simulink model "ADCtoDACloopback"  (R2015b)
settings: Solver=VariableStepAuto  StartTime=0.0  StopTime=10.0  RelTol=1e-3
undefined symbols (not defined in the file): AXI4, fClk, Lite
libraries: xbsIndex_r4 x115
settings Model: Creator=sebek  LastModifiedBy=sebek

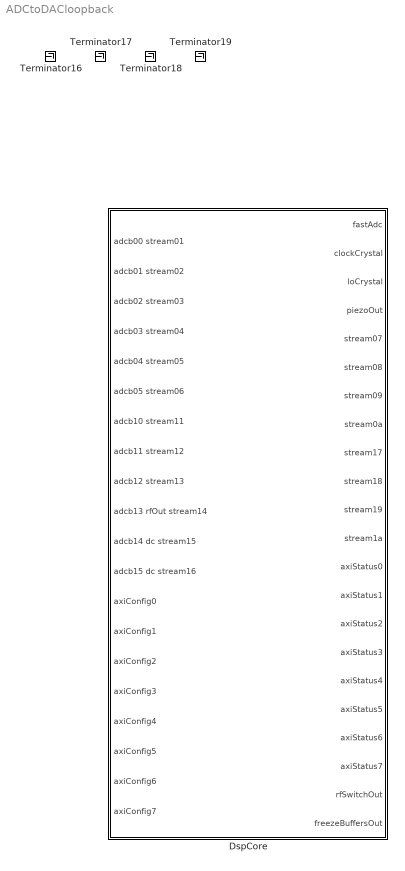
== system ADCtoDACloopback ==
  DspCore : Subsystem
  Terminator{16..19} (4 alike) : Terminator

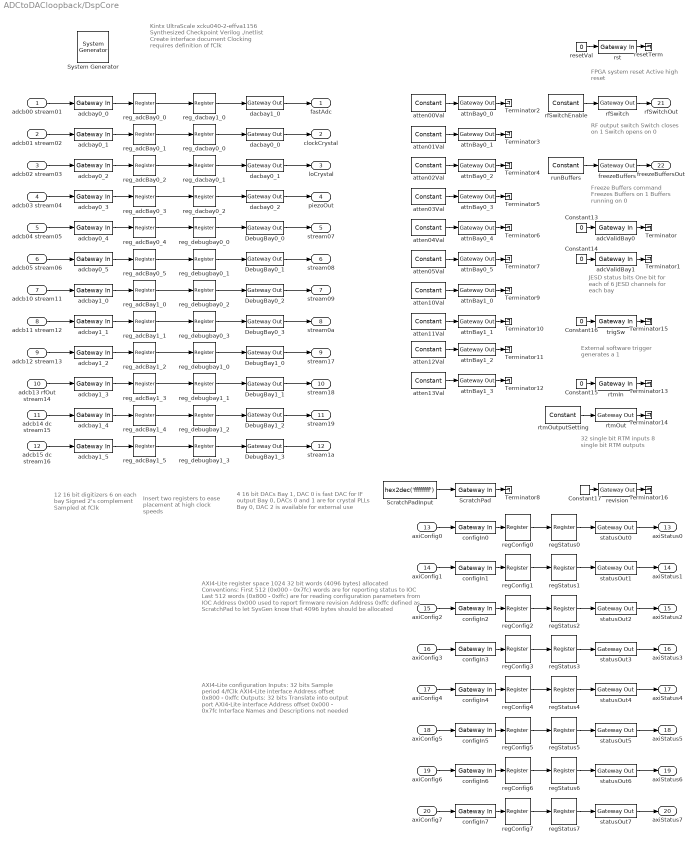
== system ADCtoDACloopback/DspCore ==
  note: AXI4-Lite configuration
      | Inputs:
      | 32 bits
      | Sample period 4/fClk
      | AXI4-Lite interface
      | Address offset 0x800 - 0xffc
      | Outputs:
      | 32 bits
      | Translate into output port
      | AXI4-Lite interface
      | Address offset 0x000 - 0x7fc
      | Interface Names and Descriptions not needed
  note: AXI4-Lite register space
      | 1024 32 bit words (4096 bytes) allocated
      | Conventions:
      | First 512 (0x000 - 0x7fc) words are for reporting status to IOC
      | Last 512 words (0x800 - 0xffc) are for reading configuration
      | parameters from IOC
      | Address 0x000 used to report firmware revision
      | Address 0xffc defined as ScratchPad to let SysGen know that
      | 4096 bytes should be allocated
  note: 32 single bit RTM inputs
      | 8 single bit RTM outputs
  note: External software trigger
      | generates a 1
  note: JESD status bits
      | One bit for each of
      | 6 JESD channels
      | for each bay
  note: RF output switch
      | Switch closes on 1
      | Switch opens on 0
  note: 4 16 bit DACs
      | Bay 1, DAC 0 is fast DAC for IF output
      | Bay 0, DACs 0 and 1 are for crystal PLLs
      | Bay 0, DAC 2 is available for external use
  note: Insert two registers
      | to ease placement
      | at high clock speeds
  note: 12 16 bit digitizers
      | 6 on each bay
      | Signed 2's complement
      | Sampled at fClk
  note: Kintx UltraScale xcku040-2-effva1156
      | Synthesized Checkpoint
      | Verilog
      | ./netlist
      | Create interface document
      | Clocking requires definition of fClk
  note: FPGA system reset
      | Active high reset
  note: Freeze Buffers command
      | Freezes Buffers on 1
      | Buffers running on 0
  adcb00 stream01 : Inport
  adcb01 stream02 : Inport  Port=2
  adcb02 stream03 : Inport  Port=3
  adcb03 stream04 : Inport  Port=4
  adcb04 stream05 : Inport  Port=5
  adcb05 stream06 : Inport  Port=6
  adcb10 stream11 : Inport  Port=7
  adcb11 stream12 : Inport  Port=8
  adcb12 stream13 : Inport  Port=9
  adcb13 rfOut stream14 : Inport  Port=10
  adcb14 dc stream15 : Inport  Port=11
  adcb15 dc stream16 : Inport  Port=12
  axiConfig0 : Inport  Port=13
  axiConfig1 : Inport  Port=14
  axiConfig2 : Inport  Port=15
  axiConfig3 : Inport  Port=16
  axiConfig4 : Inport  Port=17
  axiConfig5 : Inport  Port=18
  axiConfig6 : Inport  Port=19
  axiConfig7 : Inport  Port=20
  " System Generator" : xbsIndex_r4/ System Generator  Tag=genX  xilinxfamily=kintexu  part=xcku040  speed=-2-e  package=ffva1156  synthesis_tool=Vivado  clock_wrapper=Clock Enables  directory=./netlist  proj_type=Vivado  Synth_file=Vivado Synthesis Defaults  Impl_file=Vivado Implementation Defaults  testbench=off  simulink_period=1/fClk  sysclk_period=1/fClk*1e9  dcm_input_clock_period=10  incr_netlist=off  trim_vbits=Everywhere in SubSystem  dbl_ovrd=According to Block Masks  core_generation=According to Block Masks  run_coregen=off  deprecated_control=off  eval_field=0  block_type=sysgen
  Constant{13..16} (4 alike) : Constant  Value=0
  Constant17 : xbsIndex_r4/Constant  const=1  gui_display_data_type=Fixed-point  arith_type=Unsigned  n_bits=32  bin_pt=0  preci_type=Single  exp_width=8  frac_width=24  explicit_period=off  period=1  equ=P=C  opselect=C  inp2=PCIN>>17  opr=+  inp1=P  carry=CIN  dbl_ovrd=off  block_type=constant
  DebugBay0_{0..3} (4 alike) : xbsIndex_r4/Gateway Out  inherit_from_input=on  hdl_port=on  rows=1  columns=1  UseAsDAC=off  DACChannel='1'  interface=None  automatic_assignment=on  address_offset=hex2dec('00')  intf_name=''  intf_description=''  timing_constraint=None  locs_specified=off  LOCs={}  io_standard={}  block_type=gatewayout
  DebugBay1_{0..3} (4 alike) : xbsIndex_r4/Gateway Out  inherit_from_input=on  hdl_port=on  rows=1  columns=1  UseAsDAC=off  DACChannel='1'  interface=None  automatic_assignment=on  address_offset=hex2dec('00')  intf_name=''  intf_description=''  timing_constraint=None  locs_specified=off  LOCs={}  io_standard={}  block_type=gatewayout
  ScratchPad : xbsIndex_r4/Gateway In  gui_display_data_type=Fixed-point  arith_type=Unsigned  n_bits=32  bin_pt=0  preci_type=Single  exp_width=8  frac_width=24  rows=1  columns=1  quantization="Round  (unbiased: +/- Inf)"  overflow=Saturate  period=1  UseAsADC=off  ADCChannel='1'  interface=AXI4-Lite  automatic_assignment=off  address_offset=hex2dec('0ffc')  intf_name=''  intf_description=''  default_value=0  timing_constraint=None  locs_specified=off  LOCs={}  io_standard={}  inherit_from_input=off  hdl_port=on  dbl_ovrd=off  block_type=gatewayin
  ScratchPadInput : Constant  Value=hex2dec('ffffffff')  OutDataTypeStr=uint32
  Terminator{,1..16} (17 alike) : Terminator
  adcValidBay0 : xbsIndex_r4/Gateway In  gui_display_data_type=Fixed-point  arith_type=Unsigned  n_bits=6  bin_pt=0  preci_type=Single  exp_width=8  frac_width=24  rows=1  columns=1  quantization="Round  (unbiased: +/- Inf)"  overflow=Saturate  period=1/fClk  UseAsADC=off  ADCChannel='1'  interface=None  automatic_assignment=on  address_offset=hex2dec('00')  intf_name=''  intf_description=''  default_value=0  timing_constraint=None  locs_specified=off  LOCs={}  io_standard={}  inherit_from_input=off  hdl_port=on  dbl_ovrd=off  block_type=gatewayin
  adcValidBay1 : xbsIndex_r4/Gateway In  gui_display_data_type=Fixed-point  arith_type=Unsigned  n_bits=6  bin_pt=0  preci_type=Single  exp_width=8  frac_width=24  rows=1  columns=1  quantization="Round  (unbiased: +/- Inf)"  overflow=Saturate  period=1/fClk  UseAsADC=off  ADCChannel='1'  interface=None  automatic_assignment=on  address_offset=hex2dec('00')  intf_name=''  intf_description=''  default_value=0  timing_constraint=None  locs_specified=off  LOCs={}  io_standard={}  inherit_from_input=off  hdl_port=on  dbl_ovrd=off  block_type=gatewayin
  adcbay0_{0..5} (6 alike) : xbsIndex_r4/Gateway In  gui_display_data_type=Fixed-point  arith_type="Signed  (2's comp)"  n_bits=16  bin_pt=0  preci_type=Single  exp_width=8  frac_width=24  rows=1  columns=1  quantization="Round  (unbiased: +/- Inf)"  overflow=Saturate  period=1/fClk  UseAsADC=off  ADCChannel='1'  interface=None  automatic_assignment=on  address_offset=hex2dec('00')  intf_name=''  intf_description=''  default_value=0  timing_constraint=None  locs_specified=off  LOCs={}  io_standard={}  inherit_from_input=off  hdl_port=on  dbl_ovrd=off  block_type=gatewayin
  adcbay1_{0..5} (6 alike) : xbsIndex_r4/Gateway In  gui_display_data_type=Fixed-point  arith_type="Signed  (2's comp)"  n_bits=16  bin_pt=0  preci_type=Single  exp_width=8  frac_width=24  rows=1  columns=1  quantization="Round  (unbiased: +/- Inf)"  overflow=Saturate  period=1/fClk  UseAsADC=off  ADCChannel='1'  interface=None  automatic_assignment=on  address_offset=hex2dec('00')  intf_name=''  intf_description=''  default_value=0  timing_constraint=None  locs_specified=off  LOCs={}  io_standard={}  inherit_from_input=off  hdl_port=on  dbl_ovrd=off  block_type=gatewayin
  atten00Val : xbsIndex_r4/Constant  const=hex2dec('3f')  gui_display_data_type=Fixed-point  arith_type=Unsigned  n_bits=6  bin_pt=0  preci_type=Single  exp_width=8  frac_width=24  explicit_period=off  period=1  equ=P=C  opselect=C  inp2=PCIN>>17  opr=+  inp1=P  carry=CIN  dbl_ovrd=off  block_type=constant
  atten01Val : xbsIndex_r4/Constant  const=hex2dec('3f')  gui_display_data_type=Fixed-point  arith_type=Unsigned  n_bits=6  bin_pt=0  preci_type=Single  exp_width=8  frac_width=24  explicit_period=off  period=1  equ=P=C  opselect=C  inp2=PCIN>>17  opr=+  inp1=P  carry=CIN  dbl_ovrd=off  block_type=constant
  atten02Val : xbsIndex_r4/Constant  const=hex2dec('3f')  gui_display_data_type=Fixed-point  arith_type=Unsigned  n_bits=6  bin_pt=0  preci_type=Single  exp_width=8  frac_width=24  explicit_period=off  period=1  equ=P=C  opselect=C  inp2=PCIN>>17  opr=+  inp1=P  carry=CIN  dbl_ovrd=off  block_type=constant
  atten03Val : xbsIndex_r4/Constant  const=hex2dec('3f')  gui_display_data_type=Fixed-point  arith_type=Unsigned  n_bits=6  bin_pt=0  preci_type=Single  exp_width=8  frac_width=24  explicit_period=off  period=1  equ=P=C  opselect=C  inp2=PCIN>>17  opr=+  inp1=P  carry=CIN  dbl_ovrd=off  block_type=constant
  atten04Val : xbsIndex_r4/Constant  const=hex2dec('3f')  gui_display_data_type=Fixed-point  arith_type=Unsigned  n_bits=6  bin_pt=0  preci_type=Single  exp_width=8  frac_width=24  explicit_period=off  period=1  equ=P=C  opselect=C  inp2=PCIN>>17  opr=+  inp1=P  carry=CIN  dbl_ovrd=off  block_type=constant
  atten05Val : xbsIndex_r4/Constant  const=hex2dec('3f')  gui_display_data_type=Fixed-point  arith_type=Unsigned  n_bits=6  bin_pt=0  preci_type=Single  exp_width=8  frac_width=24  explicit_period=off  period=1  equ=P=C  opselect=C  inp2=PCIN>>17  opr=+  inp1=P  carry=CIN  dbl_ovrd=off  block_type=constant
  atten10Val : xbsIndex_r4/Constant  const=hex2dec('3f')  gui_display_data_type=Fixed-point  arith_type=Unsigned  n_bits=6  bin_pt=0  preci_type=Single  exp_width=8  frac_width=24  explicit_period=off  period=1  equ=P=C  opselect=C  inp2=PCIN>>17  opr=+  inp1=P  carry=CIN  dbl_ovrd=off  block_type=constant
  atten11Val : xbsIndex_r4/Constant  const=hex2dec('3f')  gui_display_data_type=Fixed-point  arith_type=Unsigned  n_bits=6  bin_pt=0  preci_type=Single  exp_width=8  frac_width=24  explicit_period=off  period=1  equ=P=C  opselect=C  inp2=PCIN>>17  opr=+  inp1=P  carry=CIN  dbl_ovrd=off  block_type=constant
  atten12Val : xbsIndex_r4/Constant  const=hex2dec('3f')  gui_display_data_type=Fixed-point  arith_type=Unsigned  n_bits=6  bin_pt=0  preci_type=Single  exp_width=8  frac_width=24  explicit_period=off  period=1  equ=P=C  opselect=C  inp2=PCIN>>17  opr=+  inp1=P  carry=CIN  dbl_ovrd=off  block_type=constant
  atten13Val : xbsIndex_r4/Constant  const=hex2dec('3f')  gui_display_data_type=Fixed-point  arith_type=Unsigned  n_bits=6  bin_pt=0  preci_type=Single  exp_width=8  frac_width=24  explicit_period=off  period=1  equ=P=C  opselect=C  inp2=PCIN>>17  opr=+  inp1=P  carry=CIN  dbl_ovrd=off  block_type=constant
  attnBay0_{0..5} (6 alike) : xbsIndex_r4/Gateway Out  inherit_from_input=off  hdl_port=on  rows=1  columns=1  UseAsDAC=off  DACChannel='1'  interface=None  automatic_assignment=on  address_offset=hex2dec('00')  intf_name=''  intf_description=''  timing_constraint=None  locs_specified=off  LOCs={}  io_standard={}  block_type=gatewayout
  attnBay1_{0..3} (4 alike) : xbsIndex_r4/Gateway Out  inherit_from_input=off  hdl_port=on  rows=1  columns=1  UseAsDAC=off  DACChannel='1'  interface=None  automatic_assignment=on  address_offset=hex2dec('00')  intf_name=''  intf_description=''  timing_constraint=None  locs_specified=off  LOCs={}  io_standard={}  block_type=gatewayout
  configIn0 : xbsIndex_r4/Gateway In  gui_display_data_type=Fixed-point  arith_type="Signed  (2's comp)"  n_bits=32  bin_pt=0  preci_type=Single  exp_width=8  frac_width=24  rows=1  columns=1  quantization="Round  (unbiased: +/- Inf)"  overflow=Saturate  period=4/fClk  UseAsADC=off  ADCChannel='1'  interface=AXI4-Lite  automatic_assignment=off  address_offset=hex2dec('800')  intf_name=''  intf_description=''  default_value=0  timing_constraint=None  locs_specified=off  LOCs={}  io_standard={}  inherit_from_input=off  hdl_port=on  dbl_ovrd=off  block_type=gatewayin
  configIn1 : xbsIndex_r4/Gateway In  gui_display_data_type=Fixed-point  arith_type="Signed  (2's comp)"  n_bits=32  bin_pt=0  preci_type=Single  exp_width=8  frac_width=24  rows=1  columns=1  quantization="Round  (unbiased: +/- Inf)"  overflow=Saturate  period=4/fClk  UseAsADC=off  ADCChannel='1'  interface=AXI4-Lite  automatic_assignment=off  address_offset=hex2dec('804')  intf_name=''  intf_description=''  default_value=0  timing_constraint=None  locs_specified=off  LOCs={}  io_standard={}  inherit_from_input=off  hdl_port=on  dbl_ovrd=off  block_type=gatewayin
  configIn2 : xbsIndex_r4/Gateway In  gui_display_data_type=Fixed-point  arith_type="Signed  (2's comp)"  n_bits=32  bin_pt=0  preci_type=Single  exp_width=8  frac_width=24  rows=1  columns=1  quantization="Round  (unbiased: +/- Inf)"  overflow=Saturate  period=4/fClk  UseAsADC=off  ADCChannel='1'  interface=AXI4-Lite  automatic_assignment=off  address_offset=hex2dec('808')  intf_name=''  intf_description=''  default_value=0  timing_constraint=None  locs_specified=off  LOCs={}  io_standard={}  inherit_from_input=off  hdl_port=on  dbl_ovrd=off  block_type=gatewayin
  configIn3 : xbsIndex_r4/Gateway In  gui_display_data_type=Fixed-point  arith_type="Signed  (2's comp)"  n_bits=32  bin_pt=0  preci_type=Single  exp_width=8  frac_width=24  rows=1  columns=1  quantization="Round  (unbiased: +/- Inf)"  overflow=Saturate  period=4/fClk  UseAsADC=off  ADCChannel='1'  interface=AXI4-Lite  automatic_assignment=off  address_offset=hex2dec('80C')  intf_name=''  intf_description=''  default_value=0  timing_constraint=None  locs_specified=off  LOCs={}  io_standard={}  inherit_from_input=off  hdl_port=on  dbl_ovrd=off  block_type=gatewayin
  configIn4 : xbsIndex_r4/Gateway In  gui_display_data_type=Fixed-point  arith_type="Signed  (2's comp)"  n_bits=32  bin_pt=0  preci_type=Single  exp_width=8  frac_width=24  rows=1  columns=1  quantization="Round  (unbiased: +/- Inf)"  overflow=Saturate  period=4/fClk  UseAsADC=off  ADCChannel='1'  interface=AXI4-Lite  automatic_assignment=off  address_offset=hex2dec('810')  intf_name=''  intf_description=''  default_value=0  timing_constraint=None  locs_specified=off  LOCs={}  io_standard={}  inherit_from_input=off  hdl_port=on  dbl_ovrd=off  block_type=gatewayin
  configIn5 : xbsIndex_r4/Gateway In  gui_display_data_type=Fixed-point  arith_type="Signed  (2's comp)"  n_bits=32  bin_pt=0  preci_type=Single  exp_width=8  frac_width=24  rows=1  columns=1  quantization="Round  (unbiased: +/- Inf)"  overflow=Saturate  period=4/fClk  UseAsADC=off  ADCChannel='1'  interface=AXI4-Lite  automatic_assignment=off  address_offset=hex2dec('814')  intf_name=''  intf_description=''  default_value=0  timing_constraint=None  locs_specified=off  LOCs={}  io_standard={}  inherit_from_input=off  hdl_port=on  dbl_ovrd=off  block_type=gatewayin
  configIn6 : xbsIndex_r4/Gateway In  gui_display_data_type=Fixed-point  arith_type="Signed  (2's comp)"  n_bits=32  bin_pt=0  preci_type=Single  exp_width=8  frac_width=24  rows=1  columns=1  quantization="Round  (unbiased: +/- Inf)"  overflow=Saturate  period=4/fClk  UseAsADC=off  ADCChannel='1'  interface=AXI4-Lite  automatic_assignment=off  address_offset=hex2dec('818')  intf_name=''  intf_description=''  default_value=0  timing_constraint=None  locs_specified=off  LOCs={}  io_standard={}  inherit_from_input=off  hdl_port=on  dbl_ovrd=off  block_type=gatewayin
  configIn7 : xbsIndex_r4/Gateway In  gui_display_data_type=Fixed-point  arith_type="Signed  (2's comp)"  n_bits=32  bin_pt=0  preci_type=Single  exp_width=8  frac_width=24  rows=1  columns=1  quantization="Round  (unbiased: +/- Inf)"  overflow=Saturate  period=4/fClk  UseAsADC=off  ADCChannel='1'  interface=AXI4-Lite  automatic_assignment=off  address_offset=hex2dec('81C')  intf_name=''  intf_description=''  default_value=0  timing_constraint=None  locs_specified=off  LOCs={}  io_standard={}  inherit_from_input=off  hdl_port=on  dbl_ovrd=off  block_type=gatewayin
  dacbay0_0 : xbsIndex_r4/Gateway Out  inherit_from_input=off  hdl_port=on  rows=1  columns=1  UseAsDAC=off  DACChannel='1'  interface=None  automatic_assignment=on  address_offset=hex2dec('00')  intf_name=''  intf_description=''  timing_constraint=None  locs_specified=off  LOCs={}  io_standard={}  block_type=gatewayout
  dacbay0_1 : xbsIndex_r4/Gateway Out  inherit_from_input=off  hdl_port=on  rows=1  columns=1  UseAsDAC=off  DACChannel='1'  interface=None  automatic_assignment=on  address_offset=hex2dec('00')  intf_name=''  intf_description=''  timing_constraint=None  locs_specified=off  LOCs={}  io_standard={}  block_type=gatewayout
  dacbay0_2 : xbsIndex_r4/Gateway Out  inherit_from_input=off  hdl_port=on  rows=1  columns=1  UseAsDAC=off  DACChannel='1'  interface=None  automatic_assignment=on  address_offset=hex2dec('00')  intf_name=''  intf_description=''  timing_constraint=None  locs_specified=off  LOCs={}  io_standard={}  block_type=gatewayout
  dacbay1_0 : xbsIndex_r4/Gateway Out  inherit_from_input=off  hdl_port=on  rows=1  columns=1  UseAsDAC=off  DACChannel='1'  interface=None  automatic_assignment=on  address_offset=hex2dec('00')  intf_name=''  intf_description=''  timing_constraint=None  locs_specified=off  LOCs={}  io_standard={}  block_type=gatewayout
  freezeBuffers : xbsIndex_r4/Gateway Out  inherit_from_input=off  hdl_port=on  rows=1  columns=1  UseAsDAC=off  DACChannel='1'  interface=None  automatic_assignment=on  address_offset=hex2dec('00')  intf_name=''  intf_description=''  timing_constraint=None  locs_specified=off  LOCs={}  io_standard={}  block_type=gatewayout
  regConfig{0..7} (8 alike) : xbsIndex_r4/Register  init=0  rst=off  en=off  dbl_ovrd=off  block_type=register
  regStatus{0..7} (8 alike) : xbsIndex_r4/Register  init=0  rst=off  en=off  dbl_ovrd=off  block_type=register
  reg_adcBay0_{0..5} (6 alike) : xbsIndex_r4/Register  init=0  rst=off  en=off  dbl_ovrd=off  block_type=register
  reg_adcBay1_{0..5} (6 alike) : xbsIndex_r4/Register  init=0  rst=off  en=off  dbl_ovrd=off  block_type=register
  reg_dacbay0_0 : xbsIndex_r4/Register  init=0  rst=off  en=off  dbl_ovrd=off  block_type=register
  reg_dacbay0_1 : xbsIndex_r4/Register  init=0  rst=off  en=off  dbl_ovrd=off  block_type=register
  reg_dacbay0_2 : xbsIndex_r4/Register  init=0  rst=off  en=off  dbl_ovrd=off  block_type=register
  reg_dacbay1_0 : xbsIndex_r4/Register  init=0  rst=off  en=off  dbl_ovrd=off  block_type=register
  reg_debugbay0_{0..3} (4 alike) : xbsIndex_r4/Register  init=0  rst=off  en=off  dbl_ovrd=off  block_type=register
  reg_debugbay1_{0..3} (4 alike) : xbsIndex_r4/Register  init=0  rst=off  en=off  dbl_ovrd=off  block_type=register
  resetTerm : Terminator
  resetVal : Constant  Value=0
  revision : xbsIndex_r4/Gateway Out  inherit_from_input=off  hdl_port=on  rows=1  columns=1  UseAsDAC=off  DACChannel='1'  interface=AXI4-Lite  automatic_assignment=off  address_offset=hex2dec('000')  intf_name=''  intf_description=''  timing_constraint=None  locs_specified=off  LOCs={}  io_standard={}  block_type=gatewayout
  rfSwitch : xbsIndex_r4/Gateway Out  inherit_from_input=off  hdl_port=on  rows=1  columns=1  UseAsDAC=off  DACChannel='1'  interface=None  automatic_assignment=on  address_offset=hex2dec('00')  intf_name=''  intf_description=''  timing_constraint=None  locs_specified=off  LOCs={}  io_standard={}  block_type=gatewayout
  rfSwitchEnable : xbsIndex_r4/Constant  const=1.0  gui_display_data_type=Boolean  arith_type=Boolean  n_bits=16  bin_pt=14  preci_type=Single  exp_width=8  frac_width=24  explicit_period=off  period=1  equ=P=C  opselect=C  inp2=PCIN>>17  opr=+  inp1=P  carry=CIN  dbl_ovrd=off  block_type=constant
  rst : xbsIndex_r4/Gateway In  gui_display_data_type=Boolean  arith_type=Boolean  n_bits=16  bin_pt=14  preci_type=Single  exp_width=8  frac_width=24  rows=1  columns=1  quantization="Round  (unbiased: +/- Inf)"  overflow=Saturate  period=1/fClk  UseAsADC=off  ADCChannel='1'  interface=None  automatic_assignment=on  address_offset=hex2dec('00')  intf_name=''  intf_description=''  default_value=0  timing_constraint=None  locs_specified=off  LOCs={}  io_standard={}  inherit_from_input=off  hdl_port=on  dbl_ovrd=off  block_type=gatewayin
  rtmIn : xbsIndex_r4/Gateway In  gui_display_data_type=Fixed-point  arith_type=Unsigned  n_bits=32  bin_pt=0  preci_type=Single  exp_width=8  frac_width=24  rows=1  columns=1  quantization="Round  (unbiased: +/- Inf)"  overflow=Saturate  period=1/fClk  UseAsADC=off  ADCChannel='1'  interface=None  automatic_assignment=on  address_offset=hex2dec('00')  intf_name=''  intf_description=''  default_value=0  timing_constraint=None  locs_specified=off  LOCs={}  io_standard={}  inherit_from_input=off  hdl_port=on  dbl_ovrd=off  block_type=gatewayin
  rtmOut : xbsIndex_r4/Gateway Out  inherit_from_input=off  hdl_port=on  rows=1  columns=1  UseAsDAC=off  DACChannel='1'  interface=None  automatic_assignment=on  address_offset=hex2dec('00')  intf_name=''  intf_description=''  timing_constraint=None  locs_specified=off  LOCs={}  io_standard={}  block_type=gatewayout
  rtmOutputSetting : xbsIndex_r4/Constant  const=0  gui_display_data_type=Fixed-point  arith_type=Unsigned  n_bits=8  bin_pt=0  preci_type=Single  exp_width=8  frac_width=24  explicit_period=off  period=1  equ=P=C  opselect=C  inp2=PCIN>>17  opr=+  inp1=P  carry=CIN  dbl_ovrd=off  block_type=constant
  runBuffers : xbsIndex_r4/Constant  const=0  gui_display_data_type=Boolean  arith_type=Boolean  n_bits=16  bin_pt=14  preci_type=Single  exp_width=8  frac_width=24  explicit_period=off  period=1  equ=P=C  opselect=C  inp2=PCIN>>17  opr=+  inp1=P  carry=CIN  dbl_ovrd=off  block_type=constant
  statusOut0 : xbsIndex_r4/Gateway Out  inherit_from_input=off  hdl_port=on  rows=1  columns=1  UseAsDAC=off  DACChannel='1'  interface=AXI4-Lite  automatic_assignment=off  address_offset=hex2dec('004')  intf_name=''  intf_description=''  timing_constraint=None  locs_specified=off  LOCs={}  io_standard={}  block_type=gatewayout
  statusOut1 : xbsIndex_r4/Gateway Out  inherit_from_input=off  hdl_port=on  rows=1  columns=1  UseAsDAC=off  DACChannel='1'  interface=AXI4-Lite  automatic_assignment=off  address_offset=hex2dec('008')  intf_name=''  intf_description=''  timing_constraint=None  locs_specified=off  LOCs={}  io_standard={}  block_type=gatewayout
  statusOut2 : xbsIndex_r4/Gateway Out  inherit_from_input=off  hdl_port=on  rows=1  columns=1  UseAsDAC=off  DACChannel='1'  interface=AXI4-Lite  automatic_assignment=off  address_offset=hex2dec('00c')  intf_name=''  intf_description=''  timing_constraint=None  locs_specified=off  LOCs={}  io_standard={}  block_type=gatewayout
  statusOut3 : xbsIndex_r4/Gateway Out  inherit_from_input=off  hdl_port=on  rows=1  columns=1  UseAsDAC=off  DACChannel='1'  interface=AXI4-Lite  automatic_assignment=off  address_offset=hex2dec('010')  intf_name=''  intf_description=''  timing_constraint=None  locs_specified=off  LOCs={}  io_standard={}  block_type=gatewayout
  statusOut4 : xbsIndex_r4/Gateway Out  inherit_from_input=off  hdl_port=on  rows=1  columns=1  UseAsDAC=off  DACChannel='1'  interface=AXI4-Lite  automatic_assignment=off  address_offset=hex2dec('014')  intf_name=''  intf_description=''  timing_constraint=None  locs_specified=off  LOCs={}  io_standard={}  block_type=gatewayout
  statusOut5 : xbsIndex_r4/Gateway Out  inherit_from_input=off  hdl_port=on  rows=1  columns=1  UseAsDAC=off  DACChannel='1'  interface=AXI4-Lite  automatic_assignment=off  address_offset=hex2dec('018')  intf_name=''  intf_description=''  timing_constraint=None  locs_specified=off  LOCs={}  io_standard={}  block_type=gatewayout
  statusOut6 : xbsIndex_r4/Gateway Out  inherit_from_input=off  hdl_port=on  rows=1  columns=1  UseAsDAC=off  DACChannel='1'  interface=AXI4-Lite  automatic_assignment=off  address_offset=hex2dec('01c')  intf_name=''  intf_description=''  timing_constraint=None  locs_specified=off  LOCs={}  io_standard={}  block_type=gatewayout
  statusOut7 : xbsIndex_r4/Gateway Out  inherit_from_input=off  hdl_port=on  rows=1  columns=1  UseAsDAC=off  DACChannel='1'  interface=AXI4-Lite  automatic_assignment=off  address_offset=hex2dec('020')  intf_name=''  intf_description=''  timing_constraint=None  locs_specified=off  LOCs={}  io_standard={}  block_type=gatewayout
  trigSw : xbsIndex_r4/Gateway In  gui_display_data_type=Boolean  arith_type=Boolean  n_bits=16  bin_pt=14  preci_type=Single  exp_width=8  frac_width=24  rows=1  columns=1  quantization="Round  (unbiased: +/- Inf)"  overflow=Saturate  period=1/fClk  UseAsADC=off  ADCChannel='1'  interface=None  automatic_assignment=on  address_offset=hex2dec('00')  intf_name=''  intf_description=''  default_value=0  timing_constraint=None  locs_specified=off  LOCs={}  io_standard={}  inherit_from_input=off  hdl_port=on  dbl_ovrd=off  block_type=gatewayin
  fastAdc : Outport
  clockCrystal : Outport  Port=2
  loCrystal : Outport  Port=3
  piezoOut : Outport  Port=4
  stream07 : Outport  Port=5
  stream08 : Outport  Port=6
  stream09 : Outport  Port=7
  stream0a : Outport  Port=8
  stream17 : Outport  Port=9
  stream18 : Outport  Port=10
  stream19 : Outport  Port=11
  stream1a : Outport  Port=12
  axiStatus0 : Outport  Port=13
  axiStatus1 : Outport  Port=14
  axiStatus2 : Outport  Port=15
  axiStatus3 : Outport  Port=16
  axiStatus4 : Outport  Port=17
  axiStatus5 : Outport  Port=18
  axiStatus6 : Outport  Port=19
  axiStatus7 : Outport  Port=20
  rfSwitchOut : Outport  Port=21
  freezeBuffersOut : Outport  Port=22
  wires:
  reg_adcBay0_0/1 -> reg_dacbay1_0/1
  adcbay0_0/1 -> reg_adcBay0_0/1
  reg_adcBay0_1/1 -> reg_dacbay0_0/1
  adcbay0_1/1 -> reg_adcBay0_1/1
  reg_adcBay0_2/1 -> reg_dacbay0_1/1
  adcbay0_2/1 -> reg_adcBay0_2/1
  reg_adcBay0_3/1 -> reg_dacbay0_2/1
  adcbay0_3/1 -> reg_adcBay0_3/1
  reg_adcBay0_4/1 -> reg_debugbay0_0/1
  adcbay0_4/1 -> reg_adcBay0_4/1
  reg_adcBay0_5/1 -> reg_debugbay0_1/1
  adcbay0_5/1 -> reg_adcBay0_5/1
  reg_adcBay1_0/1 -> reg_debugbay0_2/1
  adcbay1_0/1 -> reg_adcBay1_0/1
  reg_adcBay1_1/1 -> reg_debugbay0_3/1
  adcbay1_1/1 -> reg_adcBay1_1/1
  reg_adcBay1_2/1 -> reg_debugbay1_0/1
  adcbay1_2/1 -> reg_adcBay1_2/1
  reg_adcBay1_3/1 -> reg_debugbay1_1/1
  adcbay1_3/1 -> reg_adcBay1_3/1
  reg_adcBay1_4/1 -> reg_debugbay1_2/1
  adcbay1_4/1 -> reg_adcBay1_4/1
  DebugBay0_0/1 -> stream07/1
  reg_adcBay1_5/1 -> reg_debugbay1_3/1
  adcbay1_5/1 -> reg_adcBay1_5/1
  ScratchPad/1 -> Terminator8/1
  dacbay0_0/1 -> clockCrystal/1
  dacbay0_1/1 -> loCrystal/1
  dacbay0_2/1 -> piezoOut/1
  dacbay1_0/1 -> fastAdc/1
  adcb04 stream05/1 -> adcbay0_4/1
  adcb02 stream03/1 -> adcbay0_2/1
  adcb00 stream01/1 -> adcbay0_0/1
  adcb15 dc stream16/1 -> adcbay1_5/1
  adcb03 stream04/1 -> adcbay0_3/1
  adcb01 stream02/1 -> adcbay0_1/1
  adcb12 stream13/1 -> adcbay1_2/1
  adcb05 stream06/1 -> adcbay0_5/1
  adcb10 stream11/1 -> adcbay1_0/1
  adcb11 stream12/1 -> adcbay1_1/1
  DebugBay0_1/1 -> stream08/1
  DebugBay0_2/1 -> stream09/1
  DebugBay0_3/1 -> stream0a/1
  DebugBay1_0/1 -> stream17/1
  DebugBay1_1/1 -> stream18/1
  DebugBay1_2/1 -> stream19/1
  DebugBay1_3/1 -> stream1a/1
  reg_dacbay1_0/1 -> dacbay1_0/1
  rfSwitchEnable/1 -> rfSwitch/1
  rfSwitch/1 -> rfSwitchOut/1
  rtmOutputSetting/1 -> rtmOut/1
  atten00Val/1 -> attnBay0_0/1
  atten01Val/1 -> attnBay0_1/1
  atten03Val/1 -> attnBay0_3/1
  atten04Val/1 -> attnBay0_4/1
  atten05Val/1 -> attnBay0_5/1
  atten02Val/1 -> attnBay0_2/1
  atten11Val/1 -> attnBay1_1/1
  atten13Val/1 -> attnBay1_3/1
  atten10Val/1 -> attnBay1_0/1
  atten12Val/1 -> attnBay1_2/1
  Constant13/1 -> adcValidBay0/1
  adcValidBay0/1 -> Terminator/1
  Constant14/1 -> adcValidBay1/1
  adcValidBay1/1 -> Terminator1/1
  attnBay0_0/1 -> Terminator2/1
  attnBay0_1/1 -> Terminator3/1
  attnBay0_2/1 -> Terminator4/1
  attnBay0_3/1 -> Terminator5/1
  attnBay0_4/1 -> Terminator6/1
  attnBay0_5/1 -> Terminator7/1
  attnBay1_0/1 -> Terminator9/1
  attnBay1_1/1 -> Terminator10/1
  attnBay1_2/1 -> Terminator11/1
  attnBay1_3/1 -> Terminator12/1
  Constant15/1 -> rtmIn/1
  rtmIn/1 -> Terminator13/1
  rtmOut/1 -> Terminator14/1
  Constant16/1 -> trigSw/1
  trigSw/1 -> Terminator15/1
  axiConfig0/1 -> configIn0/1
  configIn0/1 -> regConfig0/1
  statusOut0/1 -> axiStatus0/1
  axiConfig1/1 -> configIn1/1
  configIn1/1 -> regConfig1/1
  statusOut1/1 -> axiStatus1/1
  axiConfig2/1 -> configIn2/1
  configIn2/1 -> regConfig2/1
  statusOut2/1 -> axiStatus2/1
  axiConfig3/1 -> configIn3/1
  configIn3/1 -> regConfig3/1
  statusOut3/1 -> axiStatus3/1
  revision/1 -> Terminator16/1
  Constant17/1 -> revision/1
  resetVal/1 -> rst/1
  rst/1 -> resetTerm/1
  adcb14 dc stream15/1 -> adcbay1_4/1
  adcb13 rfOut stream14/1 -> adcbay1_3/1
  reg_dacbay0_0/1 -> dacbay0_0/1
  reg_dacbay0_2/1 -> dacbay0_2/1
  reg_dacbay0_1/1 -> dacbay0_1/1
  reg_debugbay1_3/1 -> DebugBay1_3/1
  reg_debugbay0_0/1 -> DebugBay0_0/1
  reg_debugbay0_1/1 -> DebugBay0_1/1
  reg_debugbay0_2/1 -> DebugBay0_2/1
  reg_debugbay0_3/1 -> DebugBay0_3/1
  reg_debugbay1_0/1 -> DebugBay1_0/1
  reg_debugbay1_1/1 -> DebugBay1_1/1
  reg_debugbay1_2/1 -> DebugBay1_2/1
  regStatus0/1 -> statusOut0/1
  regConfig0/1 -> regStatus0/1
  regConfig1/1 -> regStatus1/1
  regConfig2/1 -> regStatus2/1
  regConfig3/1 -> regStatus3/1
  regStatus3/1 -> statusOut3/1
  regStatus2/1 -> statusOut2/1
  regStatus1/1 -> statusOut1/1
  axiConfig4/1 -> configIn4/1
  configIn4/1 -> regConfig4/1
  statusOut4/1 -> axiStatus4/1
  axiConfig5/1 -> configIn5/1
  configIn5/1 -> regConfig5/1
  statusOut5/1 -> axiStatus5/1
  axiConfig6/1 -> configIn6/1
  configIn6/1 -> regConfig6/1
  statusOut6/1 -> axiStatus6/1
  axiConfig7/1 -> configIn7/1
  configIn7/1 -> regConfig7/1
  statusOut7/1 -> axiStatus7/1
  regStatus4/1 -> statusOut4/1
  regConfig4/1 -> regStatus4/1
  regConfig5/1 -> regStatus5/1
  regConfig6/1 -> regStatus6/1
  regConfig7/1 -> regStatus7/1
  regStatus7/1 -> statusOut7/1
  regStatus6/1 -> statusOut6/1
  regStatus5/1 -> statusOut5/1
  runBuffers/1 -> freezeBuffers/1
  freezeBuffers/1 -> freezeBuffersOut/1
  ScratchPadInput/1 -> ScratchPad/1
